simulink subsystem "rss_PhiSensFaltDiaSens"  (R2023a)
settings: Solver=VariableStepAuto  StartTime=0.0  StopTime=10.0  RelTol=1e-3
undefined symbols (not defined in the file): ENM_TYPE_FALT, Gu16_ctPhiSensFaltConfCnt_C, Gu16_ctPhiSensFaltRcvyCnt_C
libraries: simulink x1, lib_debounce x1, lib_fault_definiteness x1
settings Model: Creator=xiaoqiang.yuan  LastModifiedBy=xiaoqiang.yuan

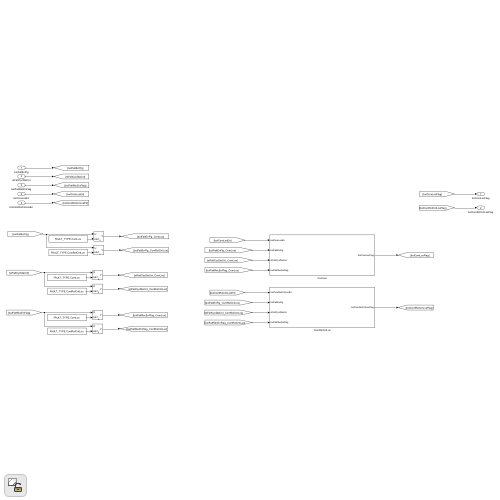
[thumbnail: Simulink's stored preview of the top-level diagram]
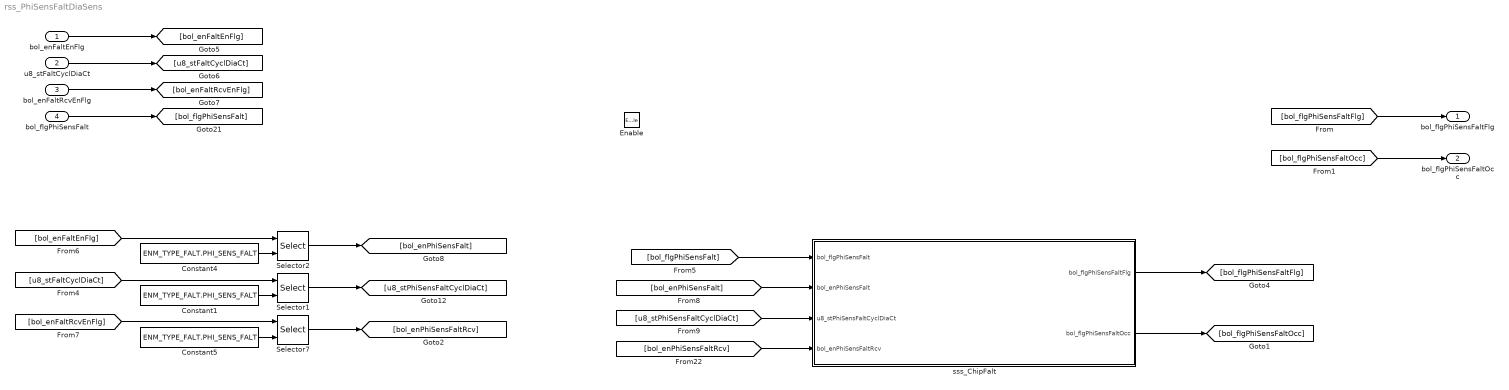
== system rss_PhiSensFaltDiaSens ==
  bol_enFaltEnFlg : Inport  OutDataTypeStr=boolean
  u8_stFaltCyclDiaCt : Inport  Port=2  OutDataTypeStr=uint8
  bol_enFaltRcvEnFlg : Inport  Port=3  OutDataTypeStr=boolean
  bol_flgPhiSensFalt : Inport  Port=4  OutDataTypeStr=boolean
  Enable : EnablePort
  Constant1 : Constant  Value=ENM_TYPE_FALT.PHI_SENS_FALT
  Constant4 : Constant  Value=ENM_TYPE_FALT.PHI_SENS_FALT
  Constant5 : Constant  Value=ENM_TYPE_FALT.PHI_SENS_FALT
  Selector1 : Selector  IndexMode=Zero-based  InputPortWidth=Cdbl_numFaltDiaNum  IndexOptions=Index vector (port)  Indices=[1 3]  OutputSizes=1
  Selector2 : Selector  IndexMode=Zero-based  InputPortWidth=Cdbl_numFaltDiaNum  IndexOptions=Index vector (port)  Indices=[1 3]  OutputSizes=1
  Selector7 : Selector  IndexMode=Zero-based  InputPortWidth=Cdbl_numFaltDiaNum  IndexOptions=Index vector (port)  Indices=[1 3]  OutputSizes=1
  sss_ChipFalt : Subsystem
  bol_flgPhiSensFaltFlg : Outport  OutDataTypeStr=boolean
  bol_flgPhiSensFaltOcc : Outport  Port=2  OutDataTypeStr=boolean
  wires:
  [bol_flgPhiSensFaltFlg] -> bol_flgPhiSensFaltFlg/1
  [u8_stFaltCyclDiaCt] -> Selector1/1
  [bol_enFaltEnFlg] -> Selector2/1
  bol_enFaltEnFlg/1 -> [bol_enFaltEnFlg]
  bol_enFaltRcvEnFlg/1 -> [bol_enFaltRcvEnFlg]
  [bol_flgPhiSensFalt] -> sss_ChipFalt/1(bol_flgPhiSensFalt)
  Constant1/1 -> Selector1/2
  [u8_stPhiSensFaltCyclDiaCt] -> sss_ChipFalt/3(u8_stPhiSensFaltCyclDiaCt)
  [bol_enPhiSensFalt] -> sss_ChipFalt/2(bol_enPhiSensFalt)
  Constant4/1 -> Selector2/2
  Constant5/1 -> Selector7/2
  Selector1/1 -> [u8_stPhiSensFaltCyclDiaCt]
  bol_flgPhiSensFalt/1 -> [bol_flgPhiSensFalt]
  Selector7/1 -> [bol_enPhiSensFaltRcv]
  [bol_enFaltRcvEnFlg] -> Selector7/1
  Selector2/1 -> [bol_enPhiSensFalt]
  [bol_enPhiSensFaltRcv] -> sss_ChipFalt/4(bol_enPhiSensFaltRcv)
  u8_stFaltCyclDiaCt/1 -> [u8_stFaltCyclDiaCt]
  sss_ChipFalt/1(bol_flgPhiSensFaltFlg) -> [bol_flgPhiSensFaltFlg]
  sss_ChipFalt/2(bol_flgPhiSensFaltOcc) -> [bol_flgPhiSensFaltOcc]
  [bol_flgPhiSensFaltOcc] -> bol_flgPhiSensFaltOcc/1

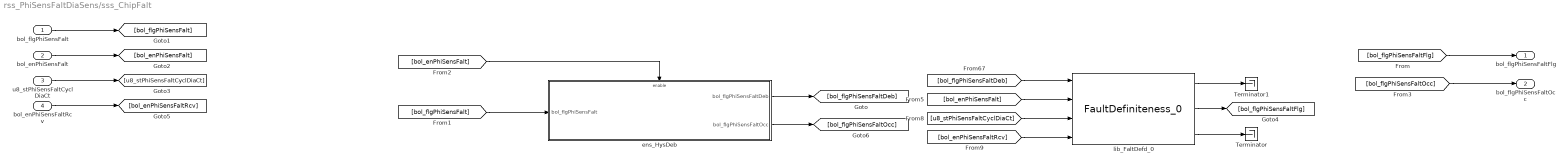
== system rss_PhiSensFaltDiaSens/sss_ChipFalt ==
  bol_flgPhiSensFalt : Inport
  bol_enPhiSensFalt : Inport  Port=2
  u8_stPhiSensFaltCyclDiaCt : Inport  Port=3
  bol_enPhiSensFaltRcv : Inport  Port=4
  Terminator : Terminator
  Terminator1 : Terminator
  ens_HysDeb : Subsystem
  lib_FaltDefd_0 : lib_fault_definiteness/FaultDefiniteness_0  lb_FaltWaitRecvCnt=Gu16_ctPhiSensFaltConfCnt_C
  bol_flgPhiSensFaltFlg : Outport
  bol_flgPhiSensFaltOcc : Outport  Port=2
  wires:
  [bol_flgPhiSensFaltOcc] -> bol_flgPhiSensFaltOcc/1
  ens_HysDeb/2(bol_flgPhiSensFaltOcc) -> [bol_flgPhiSensFaltOcc]
  lib_FaltDefd_0/1 -> Terminator1/1
  lib_FaltDefd_0/2 -> [bol_flgPhiSensFaltFlg]
  lib_FaltDefd_0/3 -> Terminator/1
  [bol_enPhiSensFalt] -> ens_HysDeb/Enable
  [bol_flgPhiSensFalt] -> ens_HysDeb/1(bol_flgPhiSensFalt)
  ens_HysDeb/1(bol_flgPhiSensFaltDeb) -> [bol_flgPhiSensFaltDeb]
  bol_enPhiSensFaltRcv/1 -> [bol_enPhiSensFaltRcv]
  u8_stPhiSensFaltCyclDiaCt/1 -> [u8_stPhiSensFaltCyclDiaCt]
  bol_enPhiSensFalt/1 -> [bol_enPhiSensFalt]
  [bol_flgPhiSensFaltFlg] -> bol_flgPhiSensFaltFlg/1
  bol_flgPhiSensFalt/1 -> [bol_flgPhiSensFalt]
  [bol_enPhiSensFaltRcv] -> lib_FaltDefd_0/4
  [u8_stPhiSensFaltCyclDiaCt] -> lib_FaltDefd_0/3
  [bol_enPhiSensFalt] -> lib_FaltDefd_0/2
  [bol_flgPhiSensFaltDeb] -> lib_FaltDefd_0/1

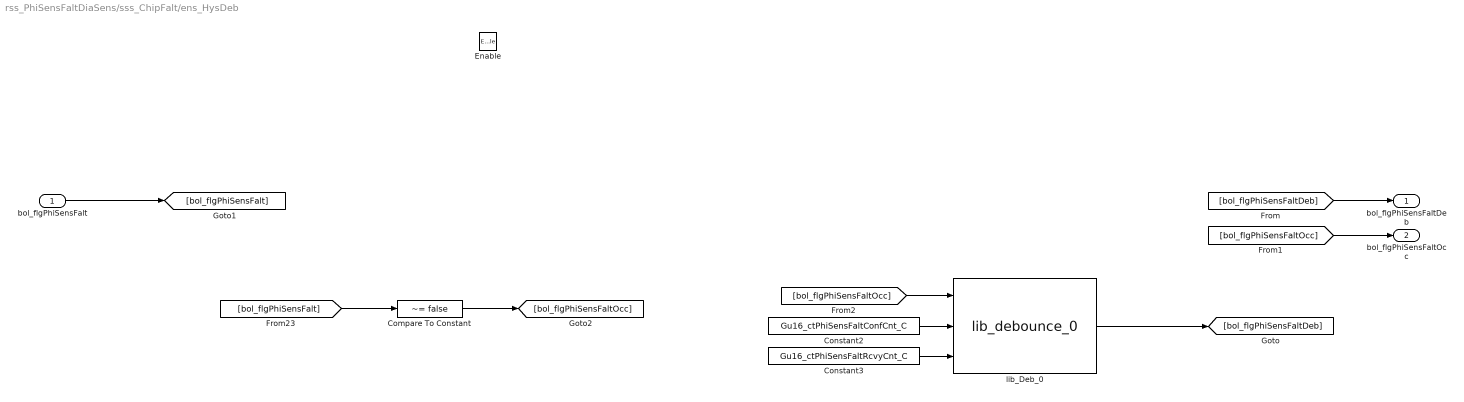
== system rss_PhiSensFaltDiaSens/sss_ChipFalt/ens_HysDeb ==
  bol_flgPhiSensFalt : Inport
  Enable : EnablePort
  Compare To Constant : simulink/Logic and Bit Operations/Compare To Constant  relop=~=  const=false  OutDataTypeStr=boolean
  Constant2 : Constant  Value=Gu16_ctPhiSensFaltConfCnt_C
  Constant3 : Constant  Value=Gu16_ctPhiSensFaltRcvyCnt_C
  lib_Deb_0 : lib_debounce/lib_debounce_0
  bol_flgPhiSensFaltDeb : Outport
  bol_flgPhiSensFaltOcc : Outport  Port=2
  wires:
  [bol_flgPhiSensFaltOcc] -> lib_Deb_0/1
  Compare To Constant/1 -> [bol_flgPhiSensFaltOcc]
  [bol_flgPhiSensFaltOcc] -> bol_flgPhiSensFaltOcc/1
  [bol_flgPhiSensFalt] -> Compare To Constant/1
  lib_Deb_0/1 -> [bol_flgPhiSensFaltDeb]
  bol_flgPhiSensFalt/1 -> [bol_flgPhiSensFalt]
  [bol_flgPhiSensFaltDeb] -> bol_flgPhiSensFaltDeb/1
  Constant3/1 -> lib_Deb_0/3
  Constant2/1 -> lib_Deb_0/2
